simulink model "overall"  (R2024a)
settings: Solver=VariableStepAuto  StartTime=0.0  StopTime=9  RelTol=1e-3
undefined symbols (not defined in the file or in its folder): Aircraft, nacelle1
libraries: simulink x1
settings Model: Creator=10335  LastModifiedBy=10335

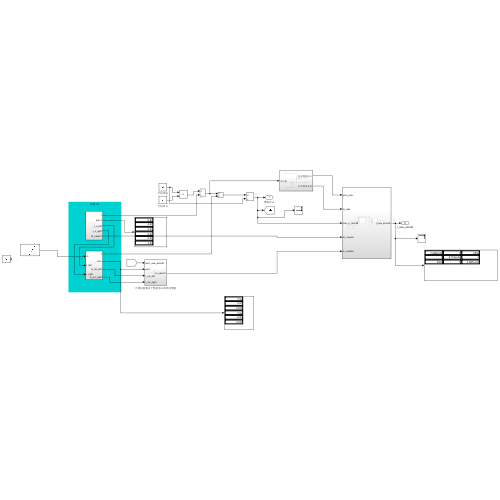
[thumbnail: Simulink's stored preview of the top-level diagram]
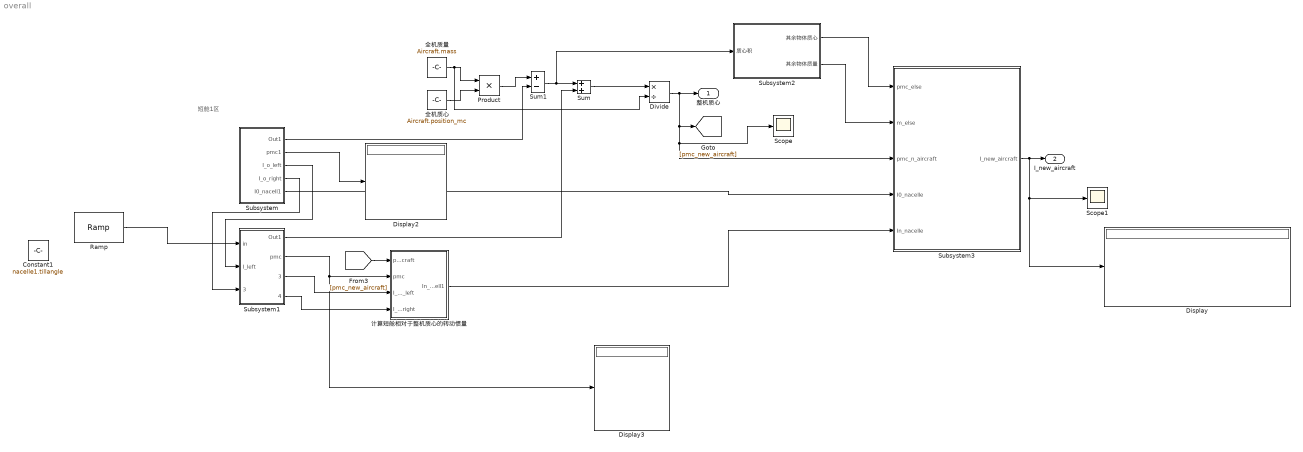
== system overall ==
  note: 短舱1区
  Constant1 : Constant  Value=nacelle1.tillangle
  Display : Display
  Display2 : Display
  Display3 : Display
  Divide : Product  Inputs=*/
  Product : Product
  Ramp : simulink/Sources/Ramp  slope=10  start=0  InitialOutput=0
  Scope : Scope
  Scope1 : Scope
  Subsystem : Subsystem
  Subsystem1 : Subsystem
  Subsystem2 : Subsystem
  Subsystem3 : Subsystem
  Sum : Sum
  Sum1 : Sum  Inputs=+-
  全机质心 : Constant  Value=Aircraft.position_mc
  全机质量 : Constant  Value=Aircraft.mass
  计算短舱相对于整机质心的转动惯量 : Subsystem
  整机质心 : Outport
  I_new_aircraft : Outport  Port=2
  wires:
  全机质量/1 -> Product/1, Divide/2
  Subsystem1/1(Out1) -> Sum/2
  Ramp/1 -> Subsystem1/1(in)
  Sum/1 -> Divide/1
  全机质心/1 -> Product/2
  Divide/1 -> [pmc_new_aircraft], Scope/1, Subsystem3/3(pmc_n_aircraft), 整机质心/1
  Subsystem/3(I_o_left) -> Subsystem1/2(I_left)
  Subsystem/4(I_o_right) -> Subsystem1/3(I_right)
  Product/1 -> Sum1/1
  Sum1/1 -> Subsystem2/1(质心积), Sum/1
  Subsystem/1(Out1) -> Sum1/2
  Subsystem2/1(其余物体质心) -> Subsystem3/1(pmc_else)
  Subsystem2/2(其余物体质量) -> Subsystem3/2(m_else)
  Subsystem3/1(I_new_aircraft) -> Scope1/1, Display/1, I_new_aircraft/1
  计算短舱相对于整机质心的转动惯量/1(In_nacell1) -> Subsystem3/5(In_nacelle)
  Subsystem1/2(pmc) -> Display3/1, 计算短舱相对于整机质心的转动惯量/2(pmc)
  Subsystem1/4(In_mc_right) -> 计算短舱相对于整机质心的转动惯量/4(I_mc_right)
  Subsystem1/3(In_mc_left) -> 计算短舱相对于整机质心的转动惯量/3(I_mc_left)
  [pmc_new_aircraft] -> 计算短舱相对于整机质心的转动惯量/1(pmc_new_aircraft)
  Subsystem/5(I0_nacell1) -> Subsystem3/4(I0_nacelle)
  Subsystem/2(pmc1) -> Display2/1

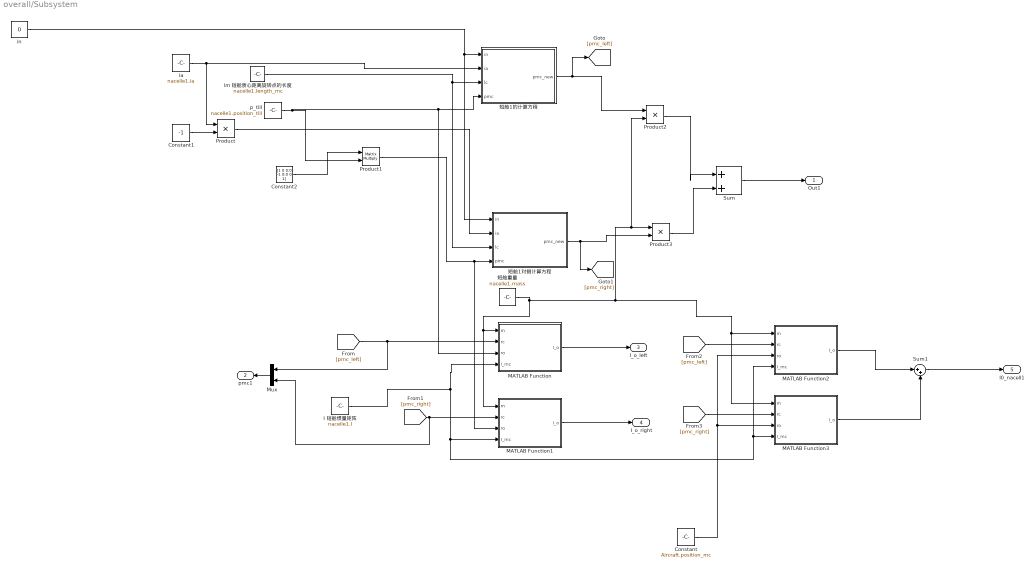
== system overall/Subsystem ==
  Constant : Constant  Value=Aircraft.position_mc
  Constant1 : Constant  Value=-1
  Constant2 : Constant  Value=[1 0 0;0 -1 0;0 0 1]
  I 短舱惯量矩阵 : Constant  Value=nacelle1.I
  MATLAB Function : MATLAB Function  TreatAsAtomicUnit=on
  MATLAB Function1 : MATLAB Function  TreatAsAtomicUnit=on
  MATLAB Function2 : MATLAB Function  TreatAsAtomicUnit=on
  MATLAB Function3 : MATLAB Function  TreatAsAtomicUnit=on
  Mux : Mux  Inputs=2
  Product : Product
  Product1 : Product  Multiplication=Matrix(*)
  Product2 : Product
  Product3 : Product
  Sum : Sum  Inputs=|++
  Sum1 : Sum  Inputs=|++
  "ia " : Constant  Value=nacelle1.ia
  in : Constant  Value=0
  lm 短舱质心距离旋转点的长度 : Constant  Value=nacelle1.length_mc
  p_till : Constant  Value=nacelle1.position_till
  短舱1对侧计算方程 : MATLAB Function  TreatAsAtomicUnit=on
  短舱1的计算方程 : MATLAB Function  TreatAsAtomicUnit=on
  短舱重量 : Constant  Value=nacelle1.mass
  Out1 : Outport
  pmc1 : Outport  Port=2
  I_o_left : Outport  Port=3
  I_o_right : Outport  Port=4
  I0_nacell1 : Outport  Port=5
  wires:
  p_till/1 -> Product1/2, MATLAB Function/3(ro), 短舱1的计算方程/4(pmc)
  Product/1 -> 短舱1对侧计算方程/2(ia)
  "ia "/1 -> Product/1, 短舱1的计算方程/2(ia)
  Constant1/1 -> Product/2
  lm 短舱质心距离旋转点的长度/1 -> 短舱1对侧计算方程/3(lc), 短舱1的计算方程/3(lc)
  in/1 -> 短舱1对侧计算方程/1(in), 短舱1的计算方程/1(in)
  Constant2/1 -> Product1/1
  Product1/1 -> MATLAB Function1/3(ro), 短舱1对侧计算方程/4(pmc)
  短舱1的计算方程/1(pmc_new) -> [pmc_left], Product2/1
  Product2/1 -> Sum/1
  短舱1对侧计算方程/1(pmc_new) -> [pmc_right], Product3/2
  Product3/1 -> Sum/2
  Sum/1 -> Out1/1
  Mux/1 -> pmc1/1
  [pmc_left] -> Mux/1, MATLAB Function/2(rc)
  [pmc_right] -> MATLAB Function1/2(rc), Mux/2
  MATLAB Function/1(I_o) -> I_o_left/1
  MATLAB Function1/1(I_o) -> I_o_right/1
  Constant/1 -> MATLAB Function2/3(ro), MATLAB Function3/3(ro)
  MATLAB Function3/1(I_o) -> Sum1/2
  MATLAB Function2/1(I_o) -> Sum1/1
  I 短舱惯量矩阵/1 -> MATLAB Function2/4(I_mc), MATLAB Function3/4(I_mc), MATLAB Function1/4(I_mc), MATLAB Function/4(I_mc)
  Sum1/1 -> I0_nacell1/1
  短舱重量/1 -> Product2/2, Product3/1, MATLAB Function3/1(m), MATLAB Function2/1(m), MATLAB Function1/1(m), MATLAB Function/1(m)
  [pmc_right] -> MATLAB Function3/2(rc)
  [pmc_left] -> MATLAB Function2/2(rc)

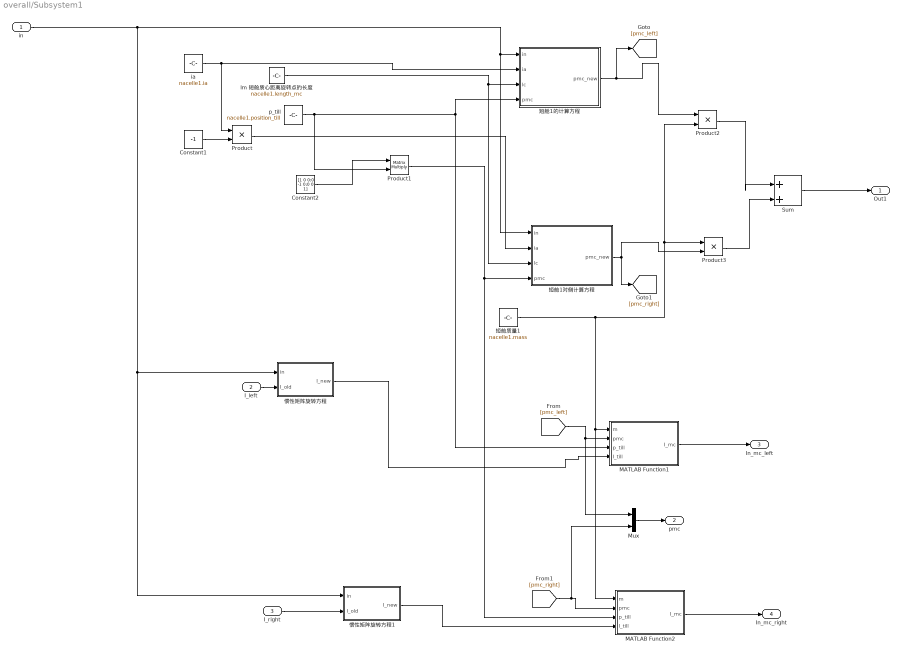
== system overall/Subsystem1 ==
  in : Inport
  I_left : Inport  Port=2
  I_right : Inport  Port=3
  Constant1 : Constant  Value=-1
  Constant2 : Constant  Value=[1 0 0;0 -1 0;0 0 1]
  MATLAB Function1 : MATLAB Function  TreatAsAtomicUnit=on
  MATLAB Function2 : MATLAB Function  TreatAsAtomicUnit=on
  Mux : Mux  Inputs=2
  Product : Product
  Product1 : Product  Multiplication=Matrix(*)
  Product2 : Product
  Product3 : Product
  Sum : Sum  Inputs=|++
  "ia " : Constant  Value=nacelle1.ia
  lm 短舱质心距离旋转点的长度 : Constant  Value=nacelle1.length_mc
  p_till : Constant  Value=nacelle1.position_till
  惯性矩阵旋转方程 : MATLAB Function  TreatAsAtomicUnit=on
  惯性矩阵旋转方程1 : MATLAB Function  TreatAsAtomicUnit=on
  短舱1对侧计算方程 : MATLAB Function  TreatAsAtomicUnit=on
  短舱1的计算方程 : MATLAB Function  TreatAsAtomicUnit=on
  短舱质量1 : Constant  Value=nacelle1.mass
  Out1 : Outport
  pmc : Outport  Port=2
  In_mc_left : Outport  Port=3
  In_mc_right : Outport  Port=4
  wires:
  Sum/1 -> Out1/1
  Product3/1 -> Sum/2
  短舱1对侧计算方程/1(pmc_new) -> [pmc_right], Product3/2
  Product2/1 -> Sum/1
  短舱1的计算方程/1(pmc_new) -> [pmc_left], Product2/1
  Product1/1 -> MATLAB Function2/3(p_till), 短舱1对侧计算方程/4(pmc)
  Constant2/1 -> Product1/1
  in/1 -> 短舱1的计算方程/1(in), 短舱1对侧计算方程/1(in), 惯性矩阵旋转方程1/1(in), 惯性矩阵旋转方程/1(in)
  lm 短舱质心距离旋转点的长度/1 -> 短舱1的计算方程/3(lc), 短舱1对侧计算方程/3(lc)
  Constant1/1 -> Product/2
  "ia "/1 -> 短舱1的计算方程/2(ia), Product/1
  Product/1 -> 短舱1对侧计算方程/2(ia)
  惯性矩阵旋转方程/1(I_new) -> MATLAB Function1/4(I_till)
  I_left/1 -> 惯性矩阵旋转方程/2(I_old)
  短舱质量1/1 -> MATLAB Function2/1(m), MATLAB Function1/1(m), Product2/2, Product3/1
  MATLAB Function1/1(I_mc) -> In_mc_left/1
  p_till/1 -> 短舱1的计算方程/4(pmc), MATLAB Function1/3(p_till), Product1/2
  I_right/1 -> 惯性矩阵旋转方程1/2(I_old)
  [pmc_left] -> Mux/1, MATLAB Function1/2(pmc)
  [pmc_right] -> Mux/2, MATLAB Function2/2(pmc)
  惯性矩阵旋转方程1/1(I_new) -> MATLAB Function2/4(I_till)
  Mux/1 -> pmc/1
  MATLAB Function2/1(I_mc) -> In_mc_right/1

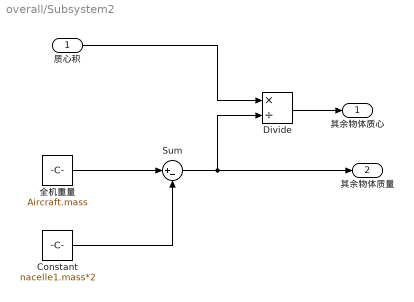
== system overall/Subsystem2 ==
  质心积 : Inport
  Constant : Constant  Value=nacelle1.mass*2
  Divide : Product  Inputs=*/
  Sum : Sum  Inputs=|+-
  全机重量 : Constant  Value=Aircraft.mass
  其余物体质心 : Outport
  其余物体质量 : Outport  Port=2
  wires:
  全机重量/1 -> Sum/1
  Constant/1 -> Sum/2
  Sum/1 -> 其余物体质量/1, Divide/2
  质心积/1 -> Divide/1
  Divide/1 -> 其余物体质心/1

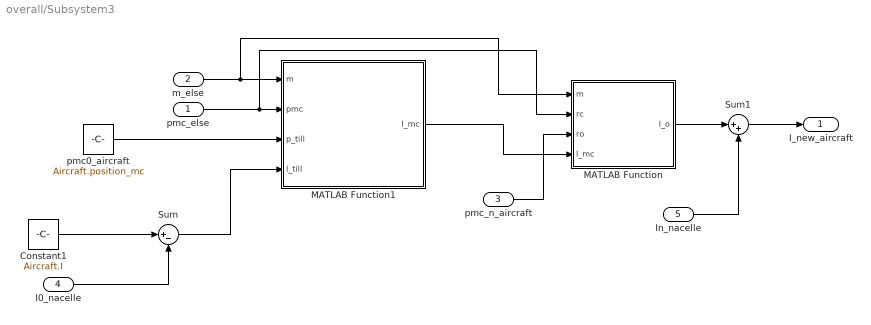
== system overall/Subsystem3 ==
  pmc_else : Inport
  m_else : Inport  Port=2
  pmc_n_aircraft : Inport  Port=3
  I0_nacelle : Inport  Port=4
  In_nacelle : Inport  Port=5
  Constant1 : Constant  Value=Aircraft.I
  MATLAB Function : MATLAB Function  TreatAsAtomicUnit=on
  MATLAB Function1 : MATLAB Function  TreatAsAtomicUnit=on
  Sum : Sum  Inputs=|+-
  Sum1 : Sum  Inputs=|++
  pmc0_aircraft : Constant  Value=Aircraft.position_mc
  I_new_aircraft : Outport
  wires:
  pmc_else/1 -> MATLAB Function/2(rc), MATLAB Function1/2(pmc)
  pmc0_aircraft/1 -> MATLAB Function1/3(p_till)
  Constant1/1 -> Sum/1
  I0_nacelle/1 -> Sum/2
  Sum/1 -> MATLAB Function1/4(I_till)
  MATLAB Function1/1(I_mc) -> MATLAB Function/4(I_mc)
  m_else/1 -> MATLAB Function/1(m), MATLAB Function1/1(m)
  pmc_n_aircraft/1 -> MATLAB Function/3(ro)
  MATLAB Function/1(I_o) -> Sum1/1
  In_nacelle/1 -> Sum1/2
  Sum1/1 -> I_new_aircraft/1

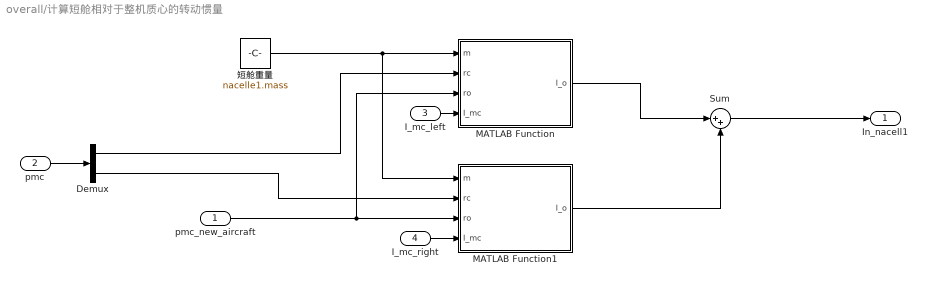
== system overall/计算短舱相对于整机质心的转动惯量 ==
  pmc_new_aircraft : Inport
  pmc : Inport  Port=2
  I_mc_left : Inport  Port=3
  I_mc_right : Inport  Port=4
  Demux : Demux  Outputs=2
  MATLAB Function : MATLAB Function  TreatAsAtomicUnit=on
  MATLAB Function1 : MATLAB Function  TreatAsAtomicUnit=on
  Sum : Sum  Inputs=|++
  短舱重量 : Constant  Value=nacelle1.mass
  In_nacell1 : Outport
  wires:
  短舱重量/1 -> MATLAB Function1/1(m), MATLAB Function/1(m)
  I_mc_left/1 -> MATLAB Function/4(I_mc)
  I_mc_right/1 -> MATLAB Function1/4(I_mc)
  pmc/1 -> Demux/1
  Demux/1 -> MATLAB Function/2(rc)
  Demux/2 -> MATLAB Function1/2(rc)
  pmc_new_aircraft/1 -> MATLAB Function/3(ro), MATLAB Function1/3(ro)
  MATLAB Function/1(I_o) -> Sum/1
  MATLAB Function1/1(I_o) -> Sum/2
  Sum/1 -> In_nacell1/1

== matlab function overall/Subsystem1/惯性矩阵旋转方程 ==
  data: in input; I_new output; I_old input
function I_new = fcn(in,I_old)
in=-in/57.3;
R=[cos(in),0,sin(in);
    0 1 0;
    -sin(in) 0 cos(in)]


I_new = R*I_old*R';

== matlab function overall/Subsystem1/惯性矩阵旋转方程1 ==
  data: in input; I_new output; I_old input
function I_new = fcn(in,I_old)
in=-in/57.3;
R=[cos(in),0,sin(in);
    0 1 0;
    -sin(in) 0 cos(in)]


I_new = R*I_old*R';

== matlab function overall/Subsystem1/MATLAB Function2 ==
  data: m input; pmc input; I_mc output; p_till input; I_till input
function I_mc = fcn(m,pmc,p_till,I_till)



x2=(p_till(1)-pmc(1))^2;
y2=(p_till(2)-pmc(2))^2;
z2=(p_till(3)-pmc(3))^2;


Ixx=I_till(1,1)-m*(y2+z2);
Iyy=I_till(2,2)-m*(x2+z2);
Izz=I_till(3,3)-m*(y2+z2);

Ixy=I_till(1,2)-m*(p_till(1)-pmc(1))*(p_till(2)-pmc(2));

Iyz=I_till(2,3)-m*(p_till(3)-pmc(3))*(p_till(2)-pmc(2));
Ixz=I_till(1,3)-m*(p_till(1)-pmc(1))*(p_till(3)-pmc(3));
I_mc = [Ixx,Ixy,Ixz;
    Ixy,Iyy,Iyz;
    Ixz,Iyz,Izz];

== matlab function overall/Subsystem/短舱1对侧计算方程 ==
  data: in input; pmc_new output; ia input; lc input; pmc input
function pmc_new  = fcn(in,ia,lc,pmc)
in=in/57.3;
pmc_new=pmc+[-lc*cos(in),lc*sin(ia),lc*cos(ia)*sin(in)]';

== matlab function overall/Subsystem3/MATLAB Function1 ==
  data: m input; pmc input; I_mc output; p_till input; I_till input
function I_mc = fcn(m,pmc,p_till,I_till)



x2=(p_till(1)-pmc(1))^2;
y2=(p_till(2)-pmc(2))^2;
z2=(p_till(3)-pmc(3))^2;


Ixx=I_till(1,1)-m*(y2+z2);
Iyy=I_till(2,2)-m*(x2+z2);
Izz=I_till(3,3)-m*(y2+z2);

Ixy=I_till(1,2)-m*(p_till(1)-pmc(1))*(p_till(2)-pmc(2));

Iyz=I_till(2,3)-m*(p_till(3)-pmc(3))*(p_till(2)-pmc(2));
Ixz=I_till(1,3)-m*(p_till(1)-pmc(1))*(p_till(3)-pmc(3));
I_mc = [Ixx,Ixy,Ixz;
    Ixy,Iyy,Iyz;
    Ixz,Iyz,Izz];

== matlab function overall/计算短舱相对于整机质心的转动惯量/MATLAB Function1 ==
  data: m input; I_o output; rc input; ro input; I_mc input
function I_o = fcn(m,rc,ro,I_mc)
x2=(rc(1)-ro(1))^2;
y2=(rc(2)-ro(2))^2;
z2=(rc(3)-ro(3))^2;


Ixx=I_mc(1,1)+m*(y2+z2);
Iyy=I_mc(2,2)+m*(x2+z2);
Izz=I_mc(3,3)+m*(y2+z2);

Ixy=I_mc(1,2)+m*(ro(1)-rc(1))*(ro(2)-rc(2));

Iyz=I_mc(2,3)+m*(ro(3)-rc(3))*(ro(2)-rc(2));
Ixz=I_mc(1,3)+m*(ro(1)-rc(1))*(ro(3)-rc(3));
I_o = [Ixx,Ixy,Ixz;
    Ixy,Iyy,Iyz;
    Ixz,Iyz,Izz];

== matlab function overall/Subsystem/MATLAB Function2 ==
  data: m input; I_o output; rc input; ro input; I_mc input
function I_o = fcn(m,rc,ro,I_mc)
x2=(rc(1)-ro(1))^2;
y2=(rc(2)-ro(2))^2;
z2=(rc(3)-ro(3))^2;


Ixx=I_mc(1,1)+m*(y2+z2);
Iyy=I_mc(2,2)+m*(x2+z2);
Izz=I_mc(3,3)+m*(y2+z2);

Ixy=I_mc(1,2)+m*(ro(1)-rc(1))*(ro(2)-rc(2));

Iyz=I_mc(2,3)+m*(ro(3)-rc(3))*(ro(2)-rc(2));
Ixz=I_mc(1,3)+m*(ro(1)-rc(1))*(ro(3)-rc(3));
I_o = [Ixx,Ixy,Ixz;
    Ixy,Iyy,Iyz;
    Ixz,Iyz,Izz];

== matlab function overall/Subsystem/MATLAB Function3 ==
  data: m input; I_o output; rc input; ro input; I_mc input
function I_o = fcn(m,rc,ro,I_mc)
x2=(rc(1)-ro(1))^2;
y2=(rc(2)-ro(2))^2;
z2=(rc(3)-ro(3))^2;


Ixx=I_mc(1,1)+m*(y2+z2);
Iyy=I_mc(2,2)+m*(x2+z2);
Izz=I_mc(3,3)+m*(y2+z2);

Ixy=I_mc(1,2)+m*(ro(1)-rc(1))*(ro(2)-rc(2));

Iyz=I_mc(2,3)+m*(ro(3)-rc(3))*(ro(2)-rc(2));
Ixz=I_mc(1,3)+m*(ro(1)-rc(1))*(ro(3)-rc(3));
I_o = [Ixx,Ixy,Ixz;
    Ixy,Iyy,Iyz;
    Ixz,Iyz,Izz];

== matlab function overall/Subsystem/短舱1的计算方程 ==
  data: in input; pmc_new output; ia input; lc input; pmc input
function pmc_new  = fcn(in,ia,lc,pmc)

in=in/57.3;
pmc_new=pmc+[-lc*cos(in),lc*sin(ia),lc*cos(ia)*sin(in)]';

== matlab function overall/Subsystem1/短舱1对侧计算方程 ==
  data: in input; pmc_new output; ia input; lc input; pmc input
function pmc_new  = fcn(in,ia,lc,pmc)
in=in/57.3;
pmc_new=pmc+[-lc*cos(in),lc*sin(ia),lc*cos(ia)*sin(in)]';

== matlab function overall/Subsystem1/短舱1的计算方程 ==
  data: in input; pmc_new output; ia input; lc input; pmc input
function pmc_new  = fcn(in,ia,lc,pmc)
in=in/57.3;
pmc_new=pmc+[-lc*cos(in),lc*sin(ia),lc*cos(ia)*sin(in)]';

== matlab function overall/Subsystem1/MATLAB Function1 ==
  data: m input; pmc input; I_mc output; p_till input; I_till input
function I_mc = fcn(m,pmc,p_till,I_till)



x2=(p_till(1)-pmc(1))^2;
y2=(p_till(2)-pmc(2))^2;
z2=(p_till(3)-pmc(3))^2;


Ixx=I_till(1,1)-m*(y2+z2);
Iyy=I_till(2,2)-m*(x2+z2);
Izz=I_till(3,3)-m*(y2+z2);

Ixy=I_till(1,2)-m*(p_till(1)-pmc(1))*(p_till(2)-pmc(2));

Iyz=I_till(2,3)-m*(p_till(3)-pmc(3))*(p_till(2)-pmc(2));
Ixz=I_till(1,3)-m*(p_till(1)-pmc(1))*(p_till(3)-pmc(3));
I_mc = [Ixx,Ixy,Ixz;
    Ixy,Iyy,Iyz;
    Ixz,Iyz,Izz];

== matlab function overall/Subsystem/MATLAB Function ==
  data: m input; I_o output; rc input; ro input; I_mc input
function I_o = fcn(m,rc,ro,I_mc)
x2=(rc(1)-ro(1))^2;
y2=(rc(2)-ro(2))^2;
z2=(rc(3)-ro(3))^2;


Ixx=I_mc(1,1)+m*(y2+z2);
Iyy=I_mc(2,2)+m*(x2+z2);
Izz=I_mc(3,3)+m*(y2+z2);

Ixy=I_mc(1,2)+m*(ro(1)-rc(1))*(ro(2)-rc(2));

Iyz=I_mc(2,3)+m*(ro(3)-rc(3))*(ro(2)-rc(2));
Ixz=I_mc(1,3)+m*(ro(1)-rc(1))*(ro(3)-rc(3));
I_o = [Ixx,Ixy,Ixz;
    Ixy,Iyy,Iyz;
    Ixz,Iyz,Izz];

== matlab function overall/Subsystem/MATLAB Function1 ==
  data: m input; I_o output; rc input; ro input; I_mc input
function I_o = fcn(m,rc,ro,I_mc)
x2=(rc(1)-ro(1))^2;
y2=(rc(2)-ro(2))^2;
z2=(rc(3)-ro(3))^2;


Ixx=I_mc(1,1)+m*(y2+z2);
Iyy=I_mc(2,2)+m*(x2+z2);
Izz=I_mc(3,3)+m*(y2+z2);

Ixy=I_mc(1,2)+m*(ro(1)-rc(1))*(ro(2)-rc(2));

Iyz=I_mc(2,3)+m*(ro(3)-rc(3))*(ro(2)-rc(2));
Ixz=I_mc(1,3)+m*(ro(1)-rc(1))*(ro(3)-rc(3));
I_o = [Ixx,Ixy,Ixz;
    Ixy,Iyy,Iyz;
    Ixz,Iyz,Izz];

== matlab function overall/计算短舱相对于整机质心的转动惯量/MATLAB Function ==
  data: m input; I_o output; rc input; ro input; I_mc input
function I_o = fcn(m,rc,ro,I_mc)
x2=(rc(1)-ro(1))^2;
y2=(rc(2)-ro(2))^2;
z2=(rc(3)-ro(3))^2;


Ixx=I_mc(1,1)+m*(y2+z2);
Iyy=I_mc(2,2)+m*(x2+z2);
Izz=I_mc(3,3)+m*(y2+z2);

Ixy=I_mc(1,2)+m*(ro(1)-rc(1))*(ro(2)-rc(2));

Iyz=I_mc(2,3)+m*(ro(3)-rc(3))*(ro(2)-rc(2));
Ixz=I_mc(1,3)+m*(ro(1)-rc(1))*(ro(3)-rc(3));
I_o = [Ixx,Ixy,Ixz;
    Ixy,Iyy,Iyz;
    Ixz,Iyz,Izz];

== matlab function overall/Subsystem3/MATLAB Function ==
  data: m input; I_o output; rc input; ro input; I_mc input
function I_o = fcn(m,rc,ro,I_mc)
x2=(rc(1)-ro(1))^2;
y2=(rc(2)-ro(2))^2;
z2=(rc(3)-ro(3))^2;


Ixx=I_mc(1,1)+m*(y2+z2);
Iyy=I_mc(2,2)+m*(x2+z2);
Izz=I_mc(3,3)+m*(y2+z2);

Ixy=I_mc(1,2)+m*(ro(1)-rc(1))*(ro(2)-rc(2));

Iyz=I_mc(2,3)+m*(ro(3)-rc(3))*(ro(2)-rc(2));
Ixz=I_mc(1,3)+m*(ro(1)-rc(1))*(ro(3)-rc(3));
I_o = [Ixx,Ixy,Ixz;
    Ixy,Iyy,Iyz;
    Ixz,Iyz,Izz];
